simulink model "sampleModel1624"  (R2023a)
settings: Solver=VariableStepAuto  StartTime=0.0  StopTime=10.0  RelTol=1e-3
libraries: simulink x2
settings Model: Creator=user1  LastModifiedBy=user1

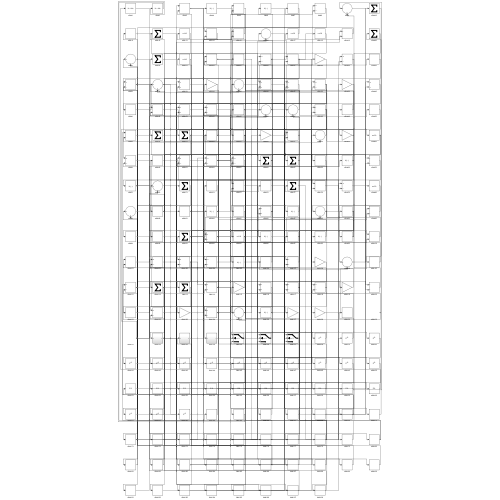
[thumbnail: Simulink's stored preview of the top-level diagram]
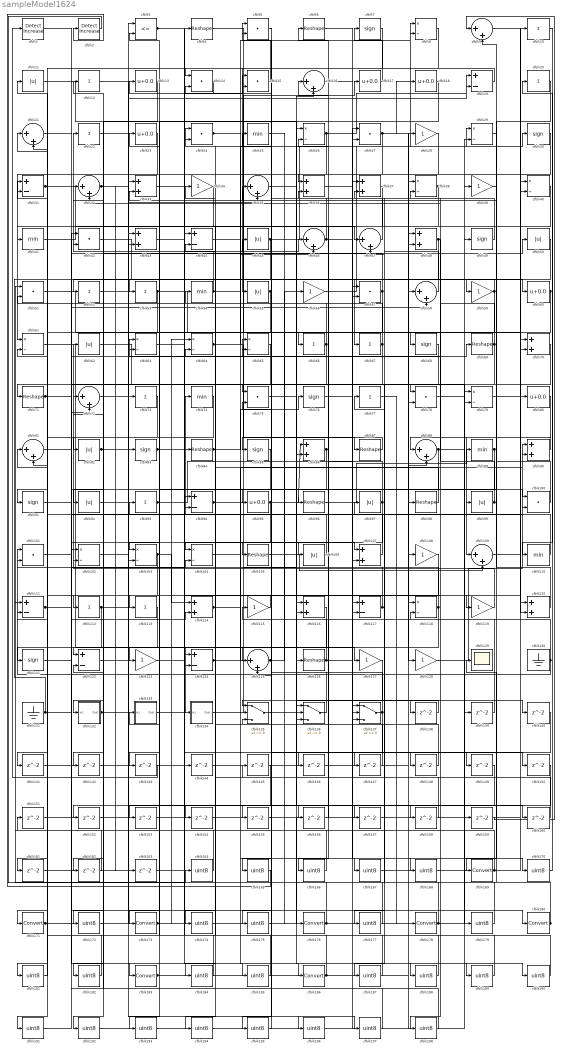
== system sampleModel1624 ==
  cfblk1 : simulink/Logic and Bit Operations/Detect Increase  vinit=0.0  OutDataTypeStr=boolean
      settings: LibrarySourceBlock=|
      | hdlsllib/Logic and Bit
      | Operations/Detect
      | Increase
  cfblk{10,12,20,22,52..53,66..67,73,77,93,112..113} (13 alike) : Sum  Inputs=+
  cfblk{5,14..15,24,27,42,51,57,75,78,100..101} (12 alike) : DotProduct  OutDataTypeStr=Inherit: Inherit via internal rule
  cfblk{8,26,29,38,40,61,63..65,79,102..104,118} (14 alike) : Product  Inputs=*/  RndMeth=Zero  SaturateOnIntegerOverflow=on
  cfblk{4,6,69,71,84,87,96,98,105,126} (10 alike) : Reshape
  cfblk{11,45,50,55,62,82,92,97,99,106} (10 alike) : Abs  SaturateOnIntegerOverflow=off
  cfblk{33,36..37,43,48,70,86,90,107,114,116,120} (12 alike) : Sum
  cfblk{28,34,39,56,59,108,115,119,123,127..128} (11 alike) : Gain
  cfblk{9,16,21,32,35,46..47,58,72,81,88,109,125} (13 alike) : Sum  Inputs=|++
  cfblk{25,41,54,74,89,110} (6 alike) : MinMax
  cfblk{19,31,44,94,111,117,122,124} (8 alike) : Sum  Inputs=+-
  cfblk{7,30,49,68,76,83,85,91,121} (9 alike) : Signum
  cfblk129 : Scope
  cfblk{13,17..18,23,60,80,95} (7 alike) : Bias  Bias=0.0  SaturateOnIntegerOverflow=off
  cfblk130 : Ground
  cfblk131 : Ground
  cfblk132 : Subsystem
      settings: LibrarySourceBlock=|
      | hdlsllib/Ports &
      | Subsystems/Subsystem
  cfblk133 : Subsystem
      settings: LibrarySourceBlock=|
      | hdlsllib/Ports &
      | Subsystems/Subsystem
  cfblk134 : Subsystem
      settings: LibrarySourceBlock=|
      | hdlsllib/Ports &
      | Subsystems/Subsystem
  cfblk135 : Switch  SaturateOnIntegerOverflow=off  InputSameDT=off
  cfblk136 : Switch  SaturateOnIntegerOverflow=off  InputSameDT=off
  cfblk137 : Switch  SaturateOnIntegerOverflow=off  InputSameDT=off
  cfblk{138..163} (26 alike) : Delay  SampleTime=1
  cfblk{164..168,170,172,174..175,177,179,181..182,184..185,187..198} (27 alike) : DataTypeConversion  OutDataTypeStr=uint8  SaturateOnIntegerOverflow=off  RndMeth=Floor
  cfblk{169,171,173,176,178,180,183,186} (8 alike) : DataTypeConversion  SaturateOnIntegerOverflow=off  RndMeth=Floor
  cfblk2 : simulink/Logic and Bit Operations/Detect Increase  vinit=0.0  OutDataTypeStr=boolean
      settings: LibrarySourceBlock=|
      | hdlsllib/Logic and Bit
      | Operations/Detect
      | Increase
  cfblk3 : RelationalOperator  Operator=<=  OutDataTypeStr=boolean  InputSameDT=off
  wires:
  cfblk125/1 -> cfblk56/1, cfblk75/2
  cfblk80/1 -> cfblk109/1
  cfblk130/1 -> cfblk101/1, cfblk115/1
  cfblk131/1 -> cfblk67/1, cfblk50/1, cfblk104/2
  cfblk44/1 -> cfblk186/1
  cfblk128/1 -> cfblk90/1
  cfblk112/1 -> cfblk122/1, cfblk19/2
  cfblk10/1 -> cfblk110/1
  cfblk134/1(Out1) -> cfblk17/1
  cfblk17/1 -> cfblk7/1
  cfblk73/1 -> cfblk171/1
  cfblk37/1 -> cfblk61/1
  cfblk136/1 -> cfblk65/1
  cfblk53/1 -> cfblk68/1, cfblk191/1
  cfblk96/1 -> cfblk89/1
  cfblk109/1 -> cfblk10/1
  cfblk95/1 -> cfblk86/1, cfblk104/1
  cfblk103/1 -> cfblk113/1, cfblk114/1
  cfblk59/1 -> cfblk53/1, cfblk156/1
  cfblk19/1 -> cfblk14/1
  cfblk23/1 -> cfblk41/1
  cfblk25/1 -> cfblk176/1
  cfblk61/1 -> cfblk134/1(In1)
  cfblk121/1 -> cfblk69/1
  cfblk94/1 -> cfblk49/1, cfblk107/2
  cfblk29/1 -> cfblk99/1
  cfblk119/1 -> cfblk62/1
  cfblk64/1 -> cfblk87/1, cfblk29/1, cfblk46/2
  cfblk54/1 -> cfblk22/1, cfblk46/1
  cfblk38/1 -> cfblk71/1, cfblk124/2, cfblk184/1
  cfblk89/1 -> cfblk136/2, cfblk153/1
  cfblk56/1 -> cfblk30/1
  cfblk116/1 -> cfblk173/1
  cfblk48/1 -> cfblk132/1(In1), cfblk125/1, cfblk198/1
  cfblk87/1 -> cfblk85/1
  cfblk4/1 -> cfblk118/1
  cfblk46/1 -> cfblk117/1, cfblk36/2
  cfblk90/1 -> cfblk88/1
  cfblk97/1 -> cfblk16/1, cfblk125/2
  cfblk107/1 -> cfblk74/1
  cfblk49/1 -> cfblk24/1
  cfblk126/1 -> cfblk65/2, cfblk140/1
  cfblk7/1 -> cfblk55/1
  cfblk27/1 -> cfblk128/1, cfblk36/1, cfblk18/1, cfblk162/1
  cfblk11/1 -> cfblk126/1
  cfblk69/1 -> cfblk92/1, cfblk32/2
  cfblk55/1 -> cfblk105/1, cfblk152/1
  cfblk20/1 -> cfblk169/1
  cfblk14/1 -> cfblk13/1
  cfblk115/1 -> cfblk112/1
  cfblk79/1 -> cfblk80/1
  cfblk57/1 -> cfblk103/1, cfblk32/1
  cfblk105/1 -> cfblk109/2
  cfblk41/1 -> cfblk47/1
  cfblk71/1 -> cfblk42/1, cfblk96/1
  cfblk22/1 -> cfblk3/1
  cfblk110/1 -> cfblk84/1
  cfblk81/1 -> cfblk180/1
  cfblk135/1 -> cfblk26/1
  cfblk43/1 -> cfblk4/1
  cfblk93/1 -> cfblk37/1, cfblk120/2, cfblk185/1
  cfblk42/1 -> cfblk108/1
  cfblk33/1 -> cfblk94/1
  cfblk111/1 -> cfblk51/2, cfblk114/2
  cfblk84/1 -> cfblk54/1, cfblk76/1
  cfblk88/1 -> cfblk39/1, cfblk157/1
  cfblk99/1 -> cfblk63/1, cfblk38/2
  cfblk30/1 -> cfblk95/1
  cfblk86/1 -> cfblk124/1, cfblk6/1
  cfblk51/1 -> cfblk120/1
  cfblk15/1 -> cfblk5/1
  cfblk132/1(Out1) -> cfblk188/1, cfblk197/1
  cfblk104/1 -> cfblk107/1
  cfblk101/1 -> cfblk93/1
  cfblk123/1 -> cfblk97/1
  cfblk16/1 -> cfblk60/1
  cfblk77/1 -> cfblk178/1
  cfblk12/1 -> cfblk100/1
  cfblk24/1 -> cfblk8/2, cfblk167/1
  cfblk1/1 -> cfblk58/2
  cfblk32/1 -> cfblk78/1, cfblk163/1
  cfblk18/1 -> cfblk123/1
  cfblk137/1 -> cfblk14/2, cfblk175/1
  cfblk52/1 -> cfblk66/1
  cfblk3/1 -> cfblk127/1, cfblk146/1
  cfblk9/1 -> cfblk70/1
  cfblk114/1 -> cfblk149/1, cfblk150/1
  cfblk118/1 -> cfblk135/2, cfblk101/2
  cfblk100/1 -> cfblk9/2
  cfblk98/1 -> cfblk34/1
  cfblk60/1 -> cfblk82/1, cfblk78/2
  cfblk8/1 -> cfblk91/1
  cfblk67/1 -> cfblk12/1, cfblk137/3
  cfblk124/1 -> cfblk16/2, cfblk90/2
  cfblk113/1 -> cfblk121/1
  cfblk21/1 -> cfblk183/1
  cfblk39/1 -> cfblk59/1
  cfblk6/1 -> cfblk119/1
  cfblk133/1(Out1) -> cfblk15/1
  cfblk82/1 -> cfblk42/2, cfblk158/1
  cfblk31/1 -> cfblk137/2, cfblk79/2
  cfblk58/1 -> cfblk33/2
  cfblk66/1 -> cfblk31/1, cfblk86/2
  cfblk47/1 -> cfblk5/2
  cfblk91/1 -> cfblk106/1
  cfblk120/1 -> cfblk35/1
  cfblk122/1 -> cfblk35/2
  cfblk106/1 -> cfblk11/1
  cfblk92/1 -> cfblk100/2
  cfblk83/1 -> cfblk45/1, cfblk15/2
  cfblk45/1 -> cfblk8/1, cfblk52/1
  cfblk26/1 -> cfblk19/1, cfblk193/1
  cfblk62/1 -> cfblk75/1
  cfblk117/1 -> cfblk3/2, cfblk147/1
  cfblk35/1 -> cfblk138/1
  cfblk138/1 -> cfblk135/1
  cfblk139/1 -> cfblk118/2
  cfblk65/1 -> cfblk141/1
  cfblk141/1 -> cfblk103/2
  cfblk13/1 -> cfblk142/1
  cfblk142/1 -> cfblk58/1
  cfblk85/1 -> cfblk143/1
  cfblk143/1 -> cfblk1/1
  cfblk63/1 -> cfblk144/1
  cfblk144/1 -> cfblk48/1
  cfblk147/1 -> cfblk135/3
  cfblk36/1 -> cfblk148/1
  cfblk148/1 -> cfblk64/2
  cfblk151/1 -> cfblk43/2
  cfblk152/1 -> cfblk70/2
  cfblk153/1 -> cfblk137/1
  cfblk68/1 -> cfblk154/1
  cfblk154/1 -> cfblk88/2
  cfblk5/1 -> cfblk155/1
  cfblk156/1 -> cfblk26/2
  cfblk157/1 -> cfblk29/2
  cfblk158/1 -> cfblk38/1
  cfblk159/1 -> cfblk9/1
  cfblk75/1 -> cfblk160/1
  cfblk160/1 -> cfblk24/2
  cfblk74/1 -> cfblk161/1
  cfblk161/1 -> cfblk33/1
  cfblk162/1 -> cfblk31/2
  cfblk163/1 -> cfblk94/2
  cfblk2/1 -> cfblk164/1
  cfblk164/1 -> cfblk23/1
  cfblk50/1 -> cfblk165/1
  cfblk165/1 -> cfblk2/1
  cfblk40/1 -> cfblk166/1
  cfblk166/1 -> cfblk43/1
  cfblk167/1 -> cfblk40/1
  cfblk146/1 -> cfblk168/1
  cfblk168/1 -> cfblk40/2
  cfblk169/1 -> cfblk151/1, cfblk111/1
  cfblk76/1 -> cfblk170/1
  cfblk170/1 -> cfblk20/1
  cfblk171/1 -> cfblk111/2, cfblk27/2, cfblk83/1
  cfblk34/1 -> cfblk172/1
  cfblk172/1 -> cfblk73/1
  cfblk173/1 -> cfblk136/3, cfblk79/1, cfblk64/1
  cfblk150/1 -> cfblk174/1
  cfblk174/1 -> cfblk116/1
  cfblk175/1 -> cfblk116/2
  cfblk176/1 -> cfblk48/2, cfblk51/1
  cfblk70/1 -> cfblk177/1
  cfblk177/1 -> cfblk25/1
  cfblk178/1 -> cfblk159/1, cfblk47/2, cfblk61/2, cfblk136/1
  cfblk78/1 -> cfblk179/1
  cfblk179/1 -> cfblk77/1
  cfblk180/1 -> cfblk37/2, cfblk129/1
  cfblk108/1 -> cfblk181/1
  cfblk181/1 -> cfblk81/1
  cfblk149/1 -> cfblk182/1
  cfblk182/1 -> cfblk81/2
  cfblk183/1 -> cfblk27/1, cfblk117/2
  cfblk184/1 -> cfblk21/1
  cfblk185/1 -> cfblk21/2
  cfblk186/1 -> cfblk122/2, cfblk63/2, cfblk98/1
  cfblk140/1 -> cfblk187/1
  cfblk187/1 -> cfblk44/1
  cfblk188/1 -> cfblk44/2
  cfblk72/1 -> cfblk189/1
  cfblk189/1 -> cfblk133/1(In1)
  cfblk155/1 -> cfblk190/1
  cfblk190/1 -> cfblk72/1
  cfblk191/1 -> cfblk72/2
  cfblk28/1 -> cfblk192/1
  cfblk192/1 -> cfblk57/1
  cfblk193/1 -> cfblk28/1
  cfblk145/1 -> cfblk194/1
  cfblk194/1 -> cfblk57/2
  cfblk127/1 -> cfblk195/1
  cfblk195/1 -> cfblk145/1
  cfblk102/1 -> cfblk196/1
  cfblk196/1 -> cfblk139/1
  cfblk197/1 -> cfblk102/1
  cfblk198/1 -> cfblk102/2

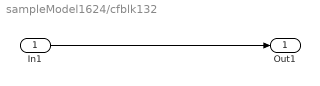
== system sampleModel1624/cfblk132 ==
  In1 : Inport
  Out1 : Outport
  wires:
  In1/1 -> Out1/1

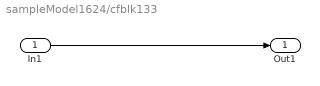
== system sampleModel1624/cfblk133 ==
  In1 : Inport
  Out1 : Outport
  wires:
  In1/1 -> Out1/1

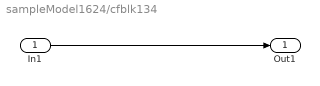
== system sampleModel1624/cfblk134 ==
  In1 : Inport
  Out1 : Outport
  wires:
  In1/1 -> Out1/1
